simulink model "ACT_Lab2_dee"  (R2018b)
settings: Solver=ode45  StartTime=0.0  StopTime=10.0  RelTol=1e-3  AbsTol=1e-6
libraries: simulink x1
settings Model: ExtModeTrigMode=oneshot  ExtModeArmWhenConnect=off  Creator=sanjai  LastModifiedBy=gaura
settings DataIOCC: SaveFormat=Array  SignalLoggingSaveFormat=ModelDataLogs  SaveOutput=off  SaveTime=off
settings OptimizationCC: BlockReduction=off  BooleanDataType=off
settings DebuggingCC: SaveWithParameterizedLinksMsg=none  UnderspecifiedInitializationDetection=Classic  MergeDetectMultiDrivingBlocksExec=none  SignalResolutionControl=TryResolveAllWithWarning  MultiTaskDSMMsg=warning  MultiTaskCondExecSysMsg=none
settings HardwareCC: TargetUnknown=on
settings ModelReferenceCC: PropagateSignalLabelsOutOfModel=off
settings GRTTargetCC: CombineOutputUpdateFcns=off  GRTInterface=on

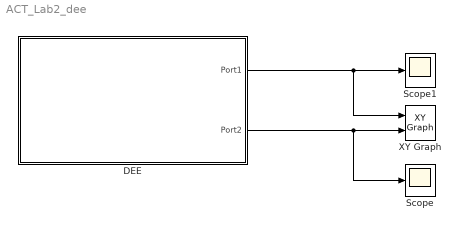
== system ACT_Lab2_dee ==
  DEE : Subsystem  mask(Differential Equation Editor (DEE)){}
      settings: OpenFcn=diffeqed
      mask Display: disp('Differential Equation\n Editor')
  Scope : Scope
  Scope1 : Scope
  XY Graph : simulink/Sinks/XY Graph  xmin=-0.2  xmax=0.2  ymin=-0.6  ymax=0.6  st=0.01
  wires:
  DEE/1(Port1) -> XY Graph/1, Scope1/1
  DEE/2(Port2) -> Scope/1, XY Graph/2

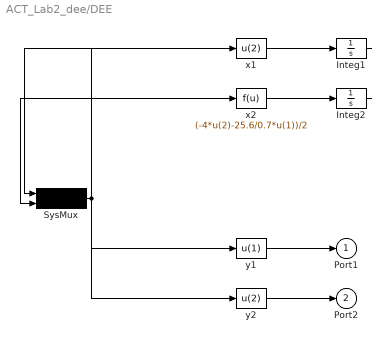
== system ACT_Lab2_dee/DEE ==
  Integ1 : Integrator
  Integ2 : Integrator  InitialCondition=0.6
  SysMux : Mux  Inputs=2
  x1 : Fcn  Expr=u(2)
  x2 : Fcn  Expr=(-4*u(2)-25.6/0.7*u(1))/2
  y1 : Fcn  Expr=u(1)
  y2 : Fcn  Expr=u(2)
  Port1 : Outport
  Port2 : Outport  Port=2
  wires:
  SysMux/1 -> x1/1, x2/1, y1/1, y2/1
  x1/1 -> Integ1/1
  Integ1/1 -> SysMux/1
  x2/1 -> Integ2/1
  Integ2/1 -> SysMux/2
  y1/1 -> Port1/1
  y2/1 -> Port2/1
